simulink model "Assignment_1"  (R2024b)
settings: Solver=VariableStepAuto  StartTime=0.0  StopTime=10.0  RelTol=1e-3
settings Model: Creator=lenovo  LastModifiedBy=girija
settings DataIOCC: Refine=5
settings OptimizationCC: ReuseModelBlockBuffer=off
settings RTWCC: GPUComputeCapability=3.5

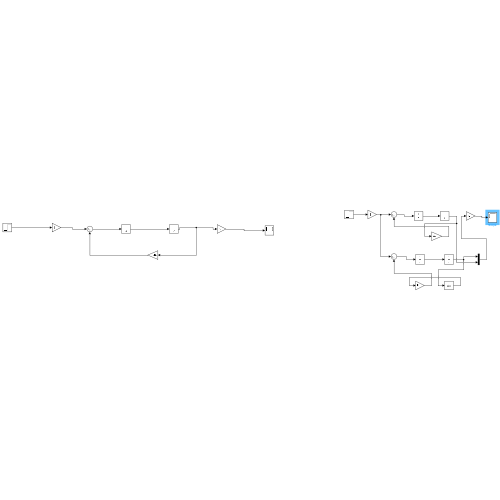
[thumbnail: Simulink's stored preview of the top-level diagram]
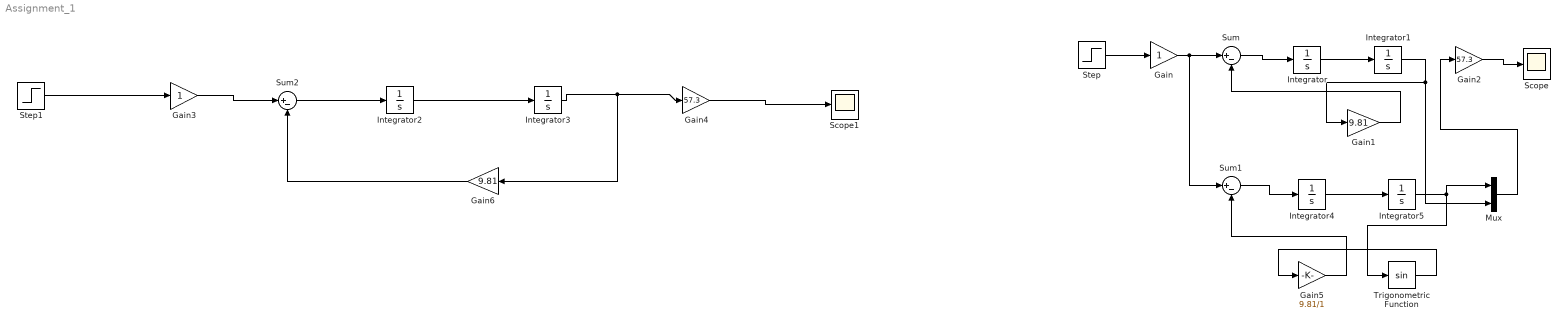
== system Assignment_1 ==
  Gain : Gain
  Gain1 : Gain  Gain=9.81
  Gain2 : Gain  Gain=57.3
  Gain3 : Gain
  Gain4 : Gain  Gain=57.3
  Gain5 : Gain  Gain=9.81/1
  Gain6 : Gain  Gain=9.81
  Integrator : Integrator
  Integrator1 : Integrator  InitialCondition=0.85
  Integrator2 : Integrator
  Integrator3 : Integrator  InitialCondition=0.85
  Integrator4 : Integrator
  Integrator5 : Integrator  InitialCondition=0.90
  Mux : Mux  Inputs=2
  Scope : Scope
  Scope1 : Scope
  Step : Step  Time=0  SampleTime=10
  Step1 : Step  Time=0  Before=2  After=2  SampleTime=10
  Sum : Sum  Inputs=|+-
  Sum1 : Sum  Inputs=|+-
  Sum2 : Sum  Inputs=|+-
  Trigonometric Function : Trigonometry
  wires:
  Step/1 -> Gain/1
  Gain/1 -> Sum1/1, Sum/1
  Sum/1 -> Integrator/1
  Integrator/1 -> Integrator1/1
  Gain2/1 -> Scope/1
  Gain1/1 -> Sum/2
  Integrator1/1 -> Mux/2, Gain1/1
  Integrator4/1 -> Integrator5/1
  Sum1/1 -> Integrator4/1
  Integrator5/1 -> Mux/1, Trigonometric Function/1
  Gain5/1 -> Sum1/2
  Trigonometric Function/1 -> Gain5/1
  Mux/1 -> Gain2/1
  Step1/1 -> Gain3/1
  Gain3/1 -> Sum2/1
  Sum2/1 -> Integrator2/1
  Integrator2/1 -> Integrator3/1
  Integrator3/1 -> Gain6/1, Gain4/1
  Gain4/1 -> Scope1/1
  Gain6/1 -> Sum2/2
